simulink model "ex_8_1"  (Simulink 10.1)
settings: Solver=VariableStepAuto  StartTime=0.0  StopTime=10.0  RelTol=1e-3
settings Model: Creator=Paulo Padrao  LastModifiedBy=Paulo Padrao
settings DataIOCC: SaveFormat=Dataset
settings OptimizationCC: LifeSpan=auto
settings DebuggingCC: UnderspecifiedInitializationDetection=Simplified  MergeDetectMultiDrivingBlocksExec=error  SFUnexpectedBacktrackingDiag=error  SFNoUnconditionalDefaultTransitionDiag=error  SFExecutionAtInitializationDiag=warning
settings HardwareCC: ProdBitPerPointer=64  ProdBitPerSizeT=64  ProdBitPerPtrDiffT=64  ProdLargestAtomicFloat=Float  ProdIntDivRoundTo=Zero  ProdEndianess=LittleEndian  ProdWordSize=64  ProdHWDeviceType=Intel->x86-64 (Windows64)
settings ModelReferenceCC: PropagateSignalLabelsOutOfModel=on
settings CodeAppCC: StateflowObjectComments=off
settings GRTTargetCC: TargetLangStandard=C99 (ISO)  CombineOutputUpdateFcns=on  GRTInterface=off
settings ConfigComp: CovMetricSettings=dwe  CovHtmlReporting=off  CovSaveCumulativeToWorkspaceVar=off  CovSaveSingleToWorkspaceVar=off  CovExternalEMLEnable=on

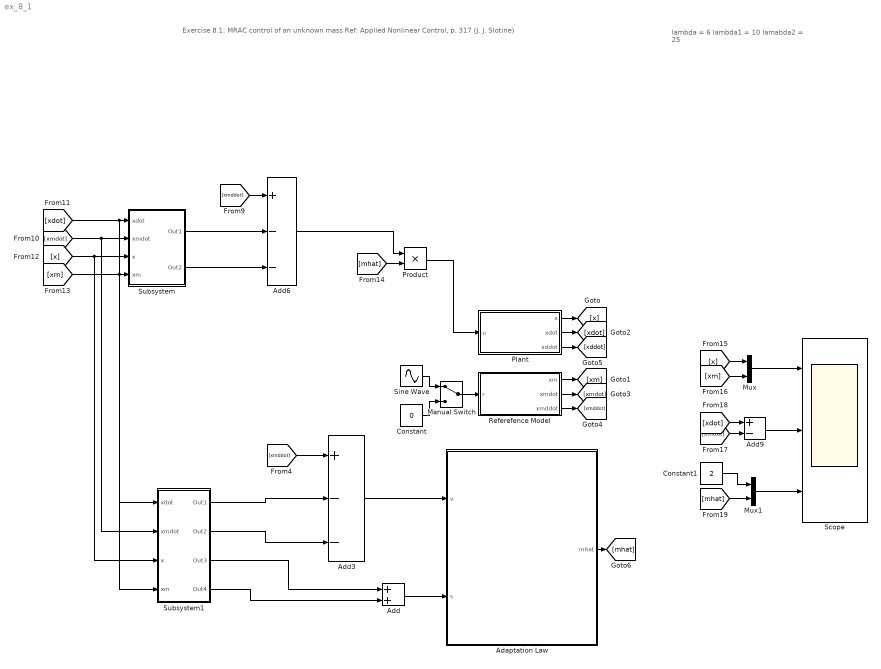
== system ex_8_1 ==
  note: Exercise 8.1: MRAC control of an unknown mass
      |
      | Ref: Applied Nonlinear Control, p. 317 (J. J. Slotine)
  note: lambda = 6
      | lambda1 = 10
      | lamabda2 = 25
  Adaptation Law : Subsystem  mask{adaptationGain=-0.5}
      mask prompts: adaptationGain "adaptation gain"
  Add : Sum
  Add3 : Sum  Inputs=+--
  Add6 : Sum  Inputs=+--
  Add9 : Sum  Inputs=+-
  Constant : Constant  Value=0
  Constant1 : Constant  Value=2
  Manual Switch : ManualSwitch
  Mux : Mux  Inputs=2
  Mux1 : Mux  Inputs=2
  Plant : Subsystem
  Product : Product
  Referefence Model : Subsystem  mask{lambda1=10, lambda2=25}
  Scope : Scope  NumInputPorts=3
  Sine Wave : Sin  Frequency=4  SampleTime=0
  Subsystem : Subsystem  mask{lambda=6}
  Subsystem1 : Subsystem  mask{lambda=6}
  wires:
  Plant/1(x) -> [x]
  Referefence Model/1(xm) -> [xm]
  Plant/2(xdot) -> [xdot]
  Referefence Model/2(xmdot) -> [xmdot]
  Add/1 -> Adaptation Law/2(s)
  Referefence Model/3(xmddot) -> [xmddot]
  Plant/3(xddot) -> [xddot]
  [xmddot] -> Add3/1
  Add3/1 -> Adaptation Law/1(v)
  Add6/1 -> Product/1
  [xmddot] -> Add6/1
  Adaptation Law/1(mhat) -> [mhat]
  [mhat] -> Product/2
  Product/1 -> Plant/1(u)
  [x] -> Mux/1
  [xm] -> Mux/2
  Mux/1 -> Scope/1
  [xdot] -> Add9/1
  [xmdot] -> Add9/2
  Add9/1 -> Scope/2
  [mhat] -> Mux1/2
  Mux1/1 -> Scope/3
  Constant1/1 -> Mux1/1
  [xdot] -> Subsystem1/1(xdot), Subsystem/1(xdot)
  [xmdot] -> Subsystem1/2(xmdot), Subsystem/2(xmdot)
  [x] -> Subsystem1/3(x), Subsystem/3(x)
  [xm] -> Subsystem1/4(xm), Subsystem/4(xm)
  Subsystem/2(Out2) -> Add6/3
  Subsystem/1(Out1) -> Add6/2
  Constant/1 -> Manual Switch/2
  Manual Switch/1 -> Referefence Model/1(r)
  Sine Wave/1 -> Manual Switch/1
  Subsystem1/1(Out1) -> Add3/2
  Subsystem1/2(Out2) -> Add3/3
  Subsystem1/3(Out3) -> Add/1
  Subsystem1/4(Out4) -> Add/2

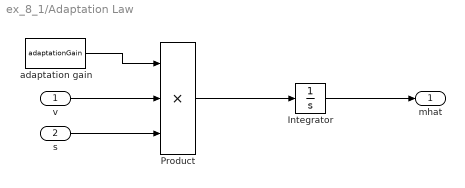
== system ex_8_1/Adaptation Law ==
  v : Inport
  s : Inport  Port=2
  Integrator : Integrator
  Product : Product  Inputs=3
  adaptation gain : Constant  Value=adaptationGain
  mhat : Outport  VectorParamsAs1DForOutWhenUnconnected=off
  wires:
  Integrator/1 -> mhat/1
  Product/1 -> Integrator/1
  adaptation gain/1 -> Product/1
  v/1 -> Product/2
  s/1 -> Product/3

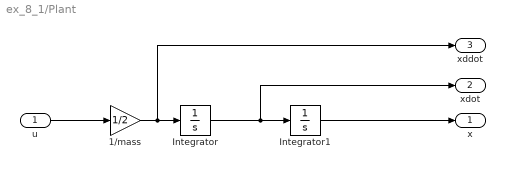
== system ex_8_1/Plant ==
  u : Inport
  1/mass : Gain  Gain=1/2
  Integrator : Integrator
  Integrator1 : Integrator  InitialCondition=0.5
  x : Outport  VectorParamsAs1DForOutWhenUnconnected=off
  xdot : Outport  Port=2  VectorParamsAs1DForOutWhenUnconnected=off
  xddot : Outport  Port=3  VectorParamsAs1DForOutWhenUnconnected=off
  wires:
  u/1 -> 1/mass/1
  Integrator/1 -> xdot/1, Integrator1/1
  Integrator1/1 -> x/1
  1/mass/1 -> xddot/1, Integrator/1

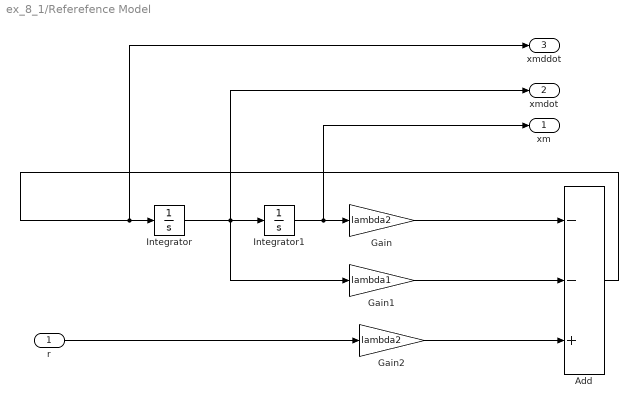
== system ex_8_1/Referefence Model ==
  r : Inport
  Add : Sum  Inputs=--+
  Gain : Gain  Gain=lambda2
  Gain1 : Gain  Gain=lambda1
  Gain2 : Gain  Gain=lambda2
  Integrator : Integrator
  Integrator1 : Integrator  InitialCondition=0.5
  xm : Outport  VectorParamsAs1DForOutWhenUnconnected=off
  xmdot : Outport  Port=2  VectorParamsAs1DForOutWhenUnconnected=off
  xmddot : Outport  Port=3  VectorParamsAs1DForOutWhenUnconnected=off
  wires:
  Integrator1/1 -> xm/1, Gain/1
  Integrator/1 -> xmdot/1, Gain1/1, Integrator1/1
  Gain/1 -> Add/1
  Gain1/1 -> Add/2
  Gain2/1 -> Add/3
  r/1 -> Gain2/1
  Add/1 -> xmddot/1, Integrator/1

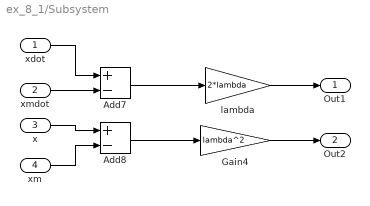
== system ex_8_1/Subsystem ==
  xdot : Inport
  xmdot : Inport  Port=2
  x : Inport  Port=3
  xm : Inport  Port=4
  Add7 : Sum  Inputs=+-
  Add8 : Sum  Inputs=+-
  Gain4 : Gain  Gain=lambda^2
  lambda : Gain  Gain=2*lambda
  Out1 : Outport
  Out2 : Outport  Port=2
  wires:
  xdot/1 -> Add7/1
  Add7/1 -> lambda/1
  lambda/1 -> Out1/1
  Add8/1 -> Gain4/1
  x/1 -> Add8/1
  xmdot/1 -> Add7/2
  Gain4/1 -> Out2/1
  xm/1 -> Add8/2

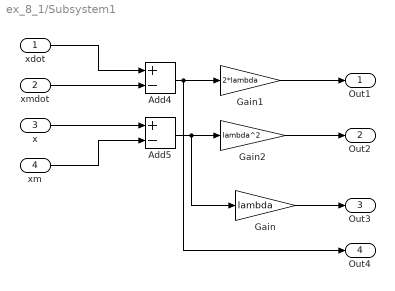
== system ex_8_1/Subsystem1 ==
  xdot : Inport
  xmdot : Inport  Port=2
  x : Inport  Port=3
  xm : Inport  Port=4
  Add4 : Sum  Inputs=+-
  Add5 : Sum  Inputs=+-
  Gain : Gain  Gain=lambda
  Gain1 : Gain  Gain=2*lambda
  Gain2 : Gain  Gain=lambda^2
  Out1 : Outport
  Out2 : Outport  Port=2
  Out3 : Outport  Port=3
  Out4 : Outport  Port=4
  wires:
  Add5/1 -> Gain/1, Gain2/1
  xm/1 -> Add5/2
  Gain/1 -> Out3/1
  Add4/1 -> Gain1/1, Out4/1
  Gain1/1 -> Out1/1
  xdot/1 -> Add4/1
  xmdot/1 -> Add4/2
  x/1 -> Add5/1
  Gain2/1 -> Out2/1
